simulink model "test_quadruped_troting"  (Simulink 9.2)
settings: Solver=VariableStepDiscrete  StartTime=0.0  StopTime=12  FixedStep=0.001  MaxStep=0.001  RelTol=1e-10  EnableMultiTasking=on
values from neighbouring files (symbols this model uses):
  Output_file_n = r_temp___(2)    [quadruped.m]
  Plant_inputs_num = r_temp___(1)    [quadruped.m]
  Plant_outputs_num = r_temp___(1)    [quadruped.m]
  RecurDyn_model_n = r_temp___(2)    [quadruped.m]
undefined symbols (not defined in the file): Matlab_version, Output_File, RecurDyn, RecurDyn_controltimestep, RecurDyn_model
(part 2 of 2)

== matlab function Subsystem/左前腿力//位控制单元 ==
  data: Th1 input double; qd input double; q input double; dot_qd input double; dot_q input double; LegMode input double; Fwd input double; Fwf input double; tau1 output double; Fr output double; Fe output double
function [tau1,Fr, Fe]  = SLC(Th1,qd,q,dot_qd,dot_q,LegMode, Fwd,Fwf)

%% 关节角度、足端广义坐标以及雅克比矩阵的计算
th11=Th1(1);
th12=Th1(2);
th13=Th1(3);

% 单腿连杆参数
L1 = 0.35*sqrt(2);
L2 = 0.35*sqrt(2);
R3 = 0.06;

% Jacobian Matrix
J1 = [ -L1*sin(th11 - th12),                   L2*sin(th12) + L1*sin(th11 - th12),                      0;...
          -L1*cos(th11 - th12)*cos(th13), -cos(th13)*(L2*cos(th12) - L1*cos(th11 - th12)), sin(th13)*(L2*sin(th12) + L1*sin(th11 - th12));...
          -L1*cos(th11 - th12)*sin(th13),  -sin(th13)*(L2*cos(th12) - L1*cos(th11 - th12)),  - cos(th13)*(L2*sin(th12) + L1*sin(th11 - th12))];

%% 初始化
 Fr=zeros(3,1);
 Fe = Fwf(1:3);    % 左前腿的足端接触力
 Fd = Fwd(1:3);
 
tau1=zeros(3,1);

%% 单腿力/位控制模式
y = LegMode;
switch(y)
%%%%%%%%%%%%%%%%%%%%%%%%%%%%%
    case 2      % 单腿支撑
        
%        p = diag([2.0  2.0  2.0]);       
%        p = diag([1.5  1.5  1.5]);
%        p = diag([1.4  1.4  1.4]);
%        p = diag([1.3  1.3  1.3]);
%        p = diag([1.2  1.2  1.2]);
       p = diag([1.1  1.1  1.1]);
%        p = diag([1.0  1.0  1.0]);
%        p = diag([0.9  0.9  0.9]);
%        p = diag([0.8  0.8  0.8]);
%        p = diag([0.7  0.7  0.7]);
%        p = diag([0.6  0.6  0.6]);
%        p = diag([0.5  0.5  0.5]);

       F=p*(Fd-Fe);
       Fr=Fd;
       
       tauf=J1'*(F+[0 Fe(2) 0]');
       tau1= -tauf;

%%%%%%%%%%%%%%%%%%%%%%%%%%%%%
    case 1    % 单腿摆动
        kp = diag([7500 7500 7500]);
        kd = diag([120 120 120]);
        
        Fr=zeros(3,1);
        tau1=J1'*(kp*(qd-q)+kd*(dot_qd-dot_q)); 
        
%%%%%%%%%%%%%%%%%%%%%%%%%%%%%
    case 0    % 落后着地
        kp = diag([1000 1500 1000]);
        kd = diag([20 30 20]);
        
        % 在y方向上补偿0.01m
        qd1= qd+[0;-0.01;0];     
        Fr=zeros(3,1);
        tau1=J1'*(kp*(qd1-q)+kd*(dot_qd-dot_q));

%%%%%%%%%%%%%%%%%%%%%%%%%%%%%
     case 3    % 提前着地
      
%        p = diag([1.2  1.2  1.2]);
       p = diag([0.8  0.8  0.8]);
       % y方向零力控制
       Fd=[0;5;0];
       F=p*(Fd-Fe);
       Fr=Fd;
       
       tauf=J1'*(F+[0 Fe(2) 0]');
       tau1=-tauf; 
end

%% 考虑实际情况：输出力矩限幅
Tmax = 500;

if tau1(1)>=Tmax
    tau1(1)=Tmax;
end
if tau1(1)<=-Tmax
    tau1(1)=-Tmax;
end
    
if tau1(2)>=Tmax
    tau1(2)=Tmax;
end
if tau1(2)<=-Tmax
    tau1(2)=-Tmax;
end
    
if tau1(3)>=Tmax
    tau1(3)=Tmax;
end
if tau1(3)<=-Tmax
    tau1(3)=-Tmax;
end

end

== matlab function 信号选择器 ==
  data: TipPos input double; HipPos output double
function HipPos  = SS(TipPos)

%% 
HipPos = TipPos(1:12);


end

== matlab function Subsystem/States Machine ==
  data: TorsoPosuture input double; VCoM input double; TipPos input double; TipForce input double; Time input double; RobotStates output double
function RobotStates   = StateMachine(TorsoPosuture, VCoM, TipPos, TipForce, Time)

% 状态机：根据当前机器人本体的状态变量 以及 足端接触力信息（作为开关量使用）， 判断并记录机器人某一特定状态及其对应的时刻
% BY ZPP
% 20171124

% TorsoPosuture：1*6（分别对应本体在世界坐标系的位置和姿态信息）
% TipForce：1*12（分别对应 左前/右前/左后/右后的足端三维力信息）
% Time：仿真时间

% RobotStates：1*35

%% 设置仿真状态初值
HipPos = TipPos(1:12);
if Time <= 0.001
    TorsoPosuture = [0; 0.70; 0;0;0;0];
    VCoM = zeros(6,1);
    HipPos = [0;-0.70;-0.0; 0;-0.70;+0.0; 0;-0.70;-0.0; 0;-0.70;+0.0];
    TipForce = zeros(12,1);
end

%% 声明局部静态变量
% 分别判断并记录四条腿TouchDown事件发生的时间点
persistent TDpoint_old1
persistent TDpoint_new1
persistent TDpoint_old2
persistent TDpoint_new2
persistent TDpoint_old3
persistent TDpoint_new3
persistent TDpoint_old4
persistent TDpoint_new4

% 分别判断并记录四条腿LiftOff事件发生的时间点
persistent LOpoint_old1
persistent LOpoint_new1
persistent LOpoint_old2
persistent LOpoint_new2
persistent LOpoint_old3
persistent LOpoint_new3
persistent LOpoint_old4
persistent LOpoint_new4

% 分别判断并记录四条腿TouchDown事件状态
persistent Swg_Sup_old1
persistent Swg_Sup_new1
persistent Swg_Sup_old2
persistent Swg_Sup_new2
persistent Swg_Sup_old3
persistent Swg_Sup_new3
persistent Swg_Sup_old4
persistent Swg_Sup_new4

% 2017/11/13增加 分别记录四条腿LiffOff事件发生时足端在髋部坐标系下的位置
persistent LOHx1_old  LOHy1_old  LOHz1_old
persistent LOHx2_old  LOHy2_old  LOHz2_old
persistent LOHx3_old  LOHy3_old  LOHz3_old
persistent LOHx4_old  LOHy4_old  LOHz4_old

persistent LOHx1_new  LOHy1_new  LOHz1_new
persistent LOHx2_new  LOHy2_new  LOHz2_new
persistent LOHx3_new  LOHy3_new  LOHz3_new
persistent LOHx4_new  LOHy4_new  LOHz4_new

% 记录本体竖直方向起跳高度以及起跳速度（所谓起跳，即四条腿均离地的那一个时刻对应的本体竖直方向高度与速度）
persistent LOTV_old
persistent LOTV_new
persistent LOTP_old
persistent LOTP_new

persistent NumTDL_old
persistent NumTDL_new

%  2017/7/19 增加  %%%%%%%%%%%%%%%%%%%%%%%%%%%%%%%%%%%
% 四足力分配模式选择（对于对角弹跳，则在【1,4】和【2,3】支撑之间选择）
persistent ForceDistMode_new
persistent ForceDistMode_old

% 2017/11/17 增加 记录力分配模式切换时间
persistent FDMSP_new
persistent FDMSP_old


% 本体在竖直方向上的位置与速度
persistent PYf_new
persistent PYf_old

% 2017/11/16新增
persistent VYf_new
persistent VYf_old

% 限制竖直方向上本体加速度切换的次数
persistent NumAccSwitch_new
persistent NumAccSwitch_old

%%%%%%%%%%%%%%%%%%%%%%%%%%%%%%%%%%%%%%%%%%%%%%

 % 变量初始化 %%%%%%%%%%%%%%%%%%%%%%%%%%%%%%%%%%%%%%
if isempty(LOTV_old)
    LOTV_old = 0;
end
if isempty(LOTV_new)
    LOTV_new = 0;
end
if isempty(LOTP_old)
    LOTP_old = 0;
end
 if isempty(LOTP_new)
    LOTP_new = 0;
 end
 
 
if isempty(NumTDL_old)
    NumTDL_old = 0;
end
 if isempty(NumTDL_new)
    NumTDL_new = 0;
end
 

if isempty(TDpoint_old1)
    TDpoint_old1 = 0;
end
if isempty(TDpoint_new1)
    TDpoint_new1 = 0;
end
if isempty(TDpoint_old2)
    TDpoint_old2 = 0;
end
if isempty(TDpoint_new2)
    TDpoint_new2 = 0;
end
if isempty(TDpoint_old3)
    TDpoint_old3 = 0;
end
if isempty(TDpoint_new3)
    TDpoint_new3 = 0;
end
if isempty(TDpoint_old4)
    TDpoint_old4 = 0;
end
if isempty(TDpoint_new4)
    TDpoint_new4 = 0;
end


if isempty(LOpoint_old1)
    LOpoint_old1 = 0;
end
if isempty(LOpoint_new1)
    LOpoint_new1 = 0;
end
if isempty(LOpoint_old2)
    LOpoint_old2 = 0;
end
if isempty(LOpoint_new2)
    LOpoint_new2 = 0;
end
if isempty(LOpoint_old3)
    LOpoint_old3 = 0;
end
if isempty(LOpoint_new3)
    LOpoint_new3 = 0;
end
if isempty(LOpoint_old4)
    LOpoint_old4 = 0;
end
if isempty(LOpoint_new4)
    LOpoint_new4 = 0;
end

%%%%%%%%%%%%%%%%%%%%%%%%%
if isempty(LOHx1_old)
    LOHx1_old = 0;
end
if isempty(LOHy1_old)
    LOHy1_old = 0;
end
if isempty(LOHz1_old)
    LOHz1_old = 0;
end

if isempty(LOHx2_old)
    LOHx2_old = 0;
end
if isempty(LOHy2_old)
    LOHy2_old = 0;
end
if isempty(LOHz2_old)
    LOHz2_old = 0;
end

if isempty(LOHx3_old)
    LOHx3_old = 0;
end
if isempty(LOHy3_old)
    LOHy3_old = 0;
end
if isempty(LOHz3_old)
    LOHz3_old = 0;
end

if isempty(LOHx4_old)
    LOHx4_old = 0;
end
if isempty(LOHy4_old)
    LOHy4_old = 0;
end
if isempty(LOHz4_old)
    LOHz4_old = 0;
end

%%%%

if isempty(LOHx1_new)
    LOHx1_new = 0;
end
if isempty(LOHy1_new)
    LOHy1_new = 0;
end
if isempty(LOHz1_new)
    LOHz1_new = 0;
end

if isempty(LOHx2_new)
    LOHx2_new = 0;
end
if isempty(LOHy2_new)
    LOHy2_new = 0;
end
if isempty(LOHz2_new)
    LOHz2_new = 0;
end

if isempty(LOHx3_new)
    LOHx3_new = 0;
end
if isempty(LOHy3_new)
    LOHy3_new = 0;
end
if isempty(LOHz3_new)
    LOHz3_new = 0;
end

if isempty(LOHx4_new)
    LOHx4_new = 0;
end
if isempty(LOHy4_new)
    LOHy4_new = 0;
end
if isempty(LOHz4_new)
    LOHz4_new = 0;
end

%%%%%%%%%%%%%%%%%%%%%%%%%

if isempty(Swg_Sup_old1)
    Swg_Sup_old1 = 0;
end
if isempty(Swg_Sup_new1)
    Swg_Sup_new1 = 0;
end
if isempty(Swg_Sup_old2)
    Swg_Sup_old2 = 0;
end
if isempty(Swg_Sup_new2)
    Swg_Sup_new2 = 0;
end
if isempty(Swg_Sup_old3)
    Swg_Sup_old3 = 0;
end
if isempty(Swg_Sup_new3)
    Swg_Sup_new3 = 0;
end
if isempty(Swg_Sup_old4)
    Swg_Sup_old4 = 0;
end
if isempty(Swg_Sup_new4)
    Swg_Sup_new4 = 0;
end


if isempty(ForceDistMode_new)
    ForceDistMode_new = 0;         % 【1】为奇数，表示为【1,4】支撑
end
if isempty(ForceDistMode_old)
    ForceDistMode_old = 0;         % 【1】为奇数，表示为【1,4】支撑
end
if isempty(FDMSP_new)
    FDMSP_new = 0;        
end
if isempty(FDMSP_old)
    FDMSP_old = 0;        
end




if isempty(PYf_new)
    PYf_new = 0;
end
if isempty(PYf_old)
    PYf_old = 0;
end

if isempty(VYf_new)
    VYf_new = 0;
end
if isempty(VYf_old)
    VYf_old = 0;
end

if isempty(NumAccSwitch_new)
    NumAccSwitch_new = 0;
end
if isempty(NumAccSwitch_old)
    NumAccSwitch_old = 0;
end


% 更新并存储上一周期和当前周期的状态值 %%%%%%%%%%%%%%%%%%%%%%%%%
lotp_old = LOTP_new;
LOTP_old = lotp_old;
lotv_old = LOTV_new;
LOTV_old = lotv_old;

numtdl_old = NumTDL_new;
NumTDL_old = numtdl_old;



tdp_old1 = TDpoint_new1;
TDpoint_old1 = tdp_old1;
tdp_old2 = TDpoint_new2;
TDpoint_old2 = tdp_old2;
tdp_old3 = TDpoint_new3;
TDpoint_old3 = tdp_old3;
tdp_old4 = TDpoint_new4;
TDpoint_old4 = tdp_old4;

lop_old1 = LOpoint_new1;
LOpoint_old1 = lop_old1;
lop_old2 = LOpoint_new2;
LOpoint_old2 = lop_old2;
lop_old3 = LOpoint_new3;
LOpoint_old3 = lop_old3;
lop_old4 = LOpoint_new4;
LOpoint_old4 = lop_old4;

%%%%%%%%%%%%%%%%%%%%%%%%
lohx1_old = LOHx1_new;
LOHx1_old = lohx1_old;
lohy1_old = LOHy1_new;
LOHy1_old = lohy1_old;
lohz1_old = LOHz1_new;
LOHz1_old = lohz1_old;

lohx2_old = LOHx2_new;
LOHx2_old = lohx2_old;
lohy2_old = LOHy2_new;
LOHy2_old = lohy2_old;
lohz2_old = LOHz2_new;
LOHz2_old = lohz2_old;

lohx3_old = LOHx3_new;
LOHx3_old = lohx3_old;
lohy3_old = LOHy3_new;
LOHy3_old = lohy3_old;
lohz3_old = LOHz3_new;
LOHz3_old = lohz3_old;

lohx4_old = LOHx4_new;
LOHx4_old = lohx4_old;
lohy4_old = LOHy4_new;
LOHy4_old = lohy4_old;
lohz4_old = LOHz4_new;
LOHz4_old = lohz4_old;

%%%%%%%%%%%%%%%%%%%%%%%%

swtotd_old1 = Swg_Sup_new1;
Swg_Sup_old1 = swtotd_old1;
swtotd_old2 = Swg_Sup_new2;
Swg_Sup_old2 = swtotd_old2;
swtotd_old3 = Swg_Sup_new3;
Swg_Sup_old3 = swtotd_old3;
swtotd_old4 = Swg_Sup_new4;
Swg_Sup_old4 = swtotd_old4;


ForceDM_old = ForceDistMode_new;
ForceDistMode_old = ForceDM_old;

fdmsp_old = FDMSP_new;
FDMSP_old = fdmsp_old;

PY_old = PYf_new;
PYf_old = PY_old;

VY_old = VYf_new;
VYf_old = VY_old;

numaccsw_old = NumAccSwitch_new;
NumAccSwitch_old = numaccsw_old;


%% 根据足端力初步判断触地状态(依此为左前/右前/左后/右后腿)  %%%%%%%%%%%%%%%%%%%%%
thre = 1;
LegState1 = (((abs(TipForce(1)))>=thre) || ((abs(TipForce(2)))>=thre) || ((abs(TipForce(3)))>=thre));  
LegState2 = (((abs(TipForce(4)))>=thre) || ((abs(TipForce(5)))>=thre) || ((abs(TipForce(6)))>=thre));  
LegState3 = (((abs(TipForce(7)))>=thre) || ((abs(TipForce(8)))>=thre) || ((abs(TipForce(9)))>=thre));  
LegState4 = (((abs(TipForce(10)))>=thre) || ((abs(TipForce(11)))>=thre) || ((abs(TipForce(12)))>=thre));  


%% 状态更新 %%%%%%%%%%%%%%%%%%%%%%%%%%%%%%%%%%%%%%%%%%%%%%

% 左前腿 %%%%%%%%%%%%%%%%%%%%%%%%%%%%%%%%%%%%%%%%%
Swg_Sup_new1 = double(LegState1);
if (Swg_Sup_new1==1) && (Swg_Sup_old1==0)
    % 由摆动向支撑切换，TouchDown事件发生的时刻得到更新
    TDpoint_new1 = Time;
     % 更新当前时刻机器人的触地状态为支撑状态
    Swg_Sup_new1 = 1;
    if ((TDpoint_new1-TDpoint_old1)<=0.05) || ((TDpoint_new1-LOpoint_new1)<=0.05)
    % 排除机器人触地瞬间在支撑期与摆动期之间高频切换（20Hz以上）
    % 否则不发生任何状态更新
    TDpoint_new1 = TDpoint_old1;
    Swg_Sup_new1 = Swg_Sup_old1;
    end
    % 但是 LiffOff 事件发生的时刻不更新
    LOpoint_new1 = LOpoint_old1;
    
elseif(Swg_Sup_new1==0) && (Swg_Sup_old1==1) 
% 同理，由支撑向摆动切换，LiffOff 事件发生的时刻得到更新
    LOpoint_new1 = Time;
    % 更新当前时刻机器人的触地状态为摆动状态
    Swg_Sup_new1 = 0;
    
    if ((LOpoint_new1-LOpoint_old1)<=0.05) || ((LOpoint_new1-TDpoint_new1)<=0.05)
        LOpoint_new1 = LOpoint_old1;
        Swg_Sup_new1 = Swg_Sup_old1;  
    end
    % 但是 TouchDown 事件发生的时刻不更新
    TDpoint_new1 = TDpoint_old1;
 
else
    % 否则不发生任何状态更新
    TDpoint_new1 = TDpoint_old1;
    LOpoint_new1 = LOpoint_old1;
    Swg_Sup_new1 = Swg_Sup_old1;  
end


% 右前腿 %%%%%%%%%%%%%%%%%%%%%%%%%%%%%%%%%%%%%%%%%
Swg_Sup_new2 = double(LegState2);
if (Swg_Sup_new2==1) && (Swg_Sup_old2==0)
    % 由摆动向支撑切换，TouchDown事件发生的时刻得到更新
    TDpoint_new2 = Time;
     % 更新当前时刻机器人的触地状态为支撑状态
    Swg_Sup_new2 = 1;
    if ((TDpoint_new2-TDpoint_old2)<=0.05) || ((TDpoint_new2-LOpoint_new2)<=0.05)
    % 排除机器人触地瞬间在支撑期与摆动期之间高频切换（100Hz以上）
    % 否则不发生任何状态更新
    TDpoint_new2 = TDpoint_old2;
    Swg_Sup_new2 = Swg_Sup_old2;
    end
    % 但是 LiffOff 事件发生的时刻不更新
    LOpoint_new2 = LOpoint_old2;
    
elseif(Swg_Sup_new2==0) && (Swg_Sup_old2==1) 
% 同理，由支撑向摆动切换，LiffOff 事件发生的时刻得到更新
    LOpoint_new2 = Time;
    % 更新当前时刻机器人的触地状态为摆动状态
    Swg_Sup_new2 = 0;
    
    if ((LOpoint_new2-LOpoint_old2)<=0.05) || ((LOpoint_new2-TDpoint_new2)<=0.05)
        LOpoint_new2 = LOpoint_old2;
        Swg_Sup_new2 = Swg_Sup_old2;  
    end
    % 但是 TouchDown 事件发生的时刻不更新
    TDpoint_new2 = TDpoint_old2;
 
else
    % 否则不发生任何状态更新
    TDpoint_new2 = TDpoint_old2;
    LOpoint_new2 = LOpoint_old2;
    Swg_Sup_new2 = Swg_Sup_old2;  
end

% 左后腿 %%%%%%%%%%%%%%%%%%%%%%%%%%%%%%%%%%%%%%%%%
Swg_Sup_new3 = double(LegState3);
if (Swg_Sup_new3==1) && (Swg_Sup_old3==0)
    % 由摆动向支撑切换，TouchDown事件发生的时刻得到更新
    TDpoint_new3 = Time;
     % 更新当前时刻机器人的触地状态为支撑状态
    Swg_Sup_new3 = 1;
    if ((TDpoint_new3-TDpoint_old3)<=0.05) || ((TDpoint_new3-LOpoint_new3)<=0.05)
    % 排除机器人触地瞬间在支撑期与摆动期之间高频切换（20Hz以上）
    % 否则不发生任何状态更新
    TDpoint_new3 = TDpoint_old3;
    Swg_Sup_new3 = Swg_Sup_old3;
    end
    % 但是 LiffOff 事件发生的时刻不更新
    LOpoint_new3 = LOpoint_old3;
    
elseif(Swg_Sup_new3==0) && (Swg_Sup_old3==1) 
% 同理，由支撑向摆动切换，LiffOff 事件发生的时刻得到更新
    LOpoint_new3 = Time;
    % 更新当前时刻机器人的触地状态为摆动状态
    Swg_Sup_new3 = 0;
    
    if ((LOpoint_new3-LOpoint_old3)<=0.05) || ((LOpoint_new3-TDpoint_new3)<=0.05)
        LOpoint_new3 = LOpoint_old3;
        Swg_Sup_new3 = Swg_Sup_old3;  
    end
    % 但是 TouchDown 事件发生的时刻不更新
    TDpoint_new3 = TDpoint_old3;
 
else
    % 否则不发生任何状态更新
    TDpoint_new3 = TDpoint_old3;
    LOpoint_new3 = LOpoint_old3;
    Swg_Sup_new3 = Swg_Sup_old3;  
end

% 右后腿%%%%%%%%%%%%%%%%%%%%%%%%%%%%%%%%%%%%%%%%%%%
Swg_Sup_new4 = double(LegState4);
if (Swg_Sup_new4==1) && (Swg_Sup_old4==0)
    % 由摆动向支撑切换，TouchDown事件发生的时刻得到更新
    TDpoint_new4 = Time;
     % 更新当前时刻机器人的触地状态为支撑状态
    Swg_Sup_new4 = 1;
    if ((TDpoint_new4-TDpoint_old4)<=0.05) || ((TDpoint_new4-LOpoint_new4)<=0.05)
    % 排除机器人触地瞬间在支撑期与摆动期之间高频切换（20Hz以上）
    % 否则不发生任何状态更新
    TDpoint_new4 = TDpoint_old4;
    Swg_Sup_new4 = Swg_Sup_old4;
    end
    % 但是 LiffOff 事件发生的时刻不更新
    LOpoint_new4 = LOpoint_old4;
    
elseif(Swg_Sup_new4==0) && (Swg_Sup_old4==1) 
% 同理，由支撑向摆动切换，LiffOff 事件发生的时刻得到更新
    LOpoint_new4 = Time;
    % 更新当前时刻机器人的触地状态为摆动状态
    Swg_Sup_new4 = 0;
    
    if ((LOpoint_new4-LOpoint_old4)<=0.05) || ((LOpoint_new4-TDpoint_new4)<=0.05)
        LOpoint_new4 = LOpoint_old4;
        Swg_Sup_new4 = Swg_Sup_old4;  
    end
    % 但是 TouchDown 事件发生的时刻不更新
    TDpoint_new4 = TDpoint_old4;
 
else
    % 否则不发生任何状态更新
    TDpoint_new4 = TDpoint_old4;
    LOpoint_new4 = LOpoint_old4;
    Swg_Sup_new4 = Swg_Sup_old4;  
end
%%%%%%%%%%%%%%%%%%%%%%%%%%%%%%%%%%%%%%%%%%%%%%%%
% Swg2Sup_old = [Swg_Sup_old1; Swg_Sup_old2; Swg_Sup_old3; Swg_Sup_old4];
Swg2Sup = [Swg_Sup_new1; Swg_Sup_new2; Swg_Sup_new3; Swg_Sup_new4];
TDP = [TDpoint_new1; TDpoint_new2; TDpoint_new3; TDpoint_new4];
LOP = [LOpoint_new1; LOpoint_new2; LOpoint_new3; LOpoint_new4];

% 稳定触地腿的数目
NumTDL = sum(sum(Swg2Sup));
% numtdl_old =  sum(sum(Swg2Sup_old));

%% 2017/11/16 限制竖直方向上本体加速度切换的次数
VYf_new = VCoM(2);
if (VYf_new >=0.40) && (VYf_old< 0.40) && (VYf_old>0.00)     % 【0.5m/s】 为本体在竖直方向上的期望起跳速度
    % 若达到期望起跳速度则切换
    NumAccSwitch_new = NumAccSwitch_old +1;
%     NumAccSwitch_new = NumAccSwitch_new
else
    % 否则不更新
    NumAccSwitch_new = NumAccSwitch_old;
end
% 进入四足腾空期，则清零
NumTDL_new = NumTDL;
if (NumTDL_new == 0)
    NumAccSwitch_new = 0;
    NumAccSwitch_old = 0;
end
numaccsw = NumAccSwitch_new;
    

%% 记录起跳时刻本体在竖直方向上的高度和速度
VyCoM = VCoM(2);
PYf = TorsoPosuture(2);

NumTDL_new = NumTDL;
% LOTP_new = PYf;
% LOTV_new = VyCoM;

if (NumTDL_new == 0) && ((NumTDL_old==2) || (NumTDL_old==1))
    % 由对角支撑期进入四足腾空期
    LOTP_new = PYf;
    LOTV_new = VyCoM;
else
    LOTP_new = LOTP_old;
    LOTV_new = LOTV_old;    
end

LOTPy = LOTP_new;
LOTVy = LOTV_new;


%% 力分配模式切换  以及 LiffOff 事件发生时刻足端在髋部坐标系下的位置

PYf_new = PYf;

if (PYf_new>=0.65) && (PYf_old<0.65)  % 【0.65】 表示腿长在【0.75m】的时候本体腾空
    % 完成一个弹跳周期进入腾空期，则四足机器人对角腿支撑进行交换，力分配模式变量得到更新
    ForceDistMode_new = ForceDistMode_old + 1;
    FDMSP_new = Time;
    % 若完成一次弹跳，则加速度切换次数清零

    %%%%%%%%%%%%%%%%%%%%%%%%%%%%%%%%%%%%%%%%%%%%%%%%%
    temp = mod(ForceDistMode_new,2);    % 奇数表示当前进入【1,4】腿支撑，偶数表示当前进入【2,3】腿支撑
    if (temp==0)  
        % Update【1,4】
        LOHx1_new = HipPos(1);  LOHy1_new = HipPos(2);  LOHz1_new = HipPos(3);
        LOHx4_new = HipPos(10);  LOHy4_new = HipPos(11);  LOHz4_new = HipPos(12);
        % maintain【2,3】
        LOHx2_new = LOHx2_old;  LOHy2_new = LOHy2_old;  LOHz2_new = LOHz2_old;
        LOHx3_new = LOHx3_old;  LOHy3_new = LOHy3_old;  LOHz3_new = LOHz3_old;
    else
        % Update【2,3】
        LOHx2_new = HipPos(4);  LOHy2_new = HipPos(5);  LOHz2_new = HipPos(6);
        LOHx3_new = HipPos(7);  LOHy3_new = HipPos(8);  LOHz3_new = HipPos(9);
        % maintain【1,4】
        LOHx1_new = LOHx1_old;  LOHy1_new = LOHy1_old;  LOHz1_new = LOHz1_old;
        LOHx4_new = LOHx4_old;  LOHy4_new = LOHy4_old;  LOHz4_new = LOHz4_old;
    end
    %%%%%%%%%%%%%%%%%%%%%%%%%%%%%%%%%%%%%%%%%%%%%%%%%    
else
    % 否则不更新
    ForceDistMode_new = ForceDistMode_old;
    FDMSP_new = FDMSP_old;
%     NumAccSwitch_new = NumAccSwitch_old;
    % maintain【1,4 & 2,3】
    LOHx1_new = LOHx1_old;  LOHy1_new = LOHy1_old;  LOHz1_new = LOHz1_old;
    LOHx4_new = LOHx4_old;  LOHy4_new = LOHy4_old;  LOHz4_new = LOHz4_old;
    LOHx2_new = LOHx2_old;  LOHy2_new = LOHy2_old;  LOHz2_new = LOHz2_old;
    LOHx3_new = LOHx3_old;  LOHy3_new = LOHy3_old;  LOHz3_new = LOHz3_old;
end

% 力分配模式：奇数为【1,4】腿支撑，偶数为【2,3】腿支撑
FDMode = mod(ForceDistMode_new,2);
FDMSP = FDMSP_new;
% 单腿LiffOff事件时刻足端在髋部坐标系下的位置
LOHipPos = [LOHx1_new; LOHy1_new; LOHz1_new; LOHx2_new; LOHy2_new; LOHz2_new; LOHx3_new; LOHy3_new; LOHz3_new; LOHx4_new; LOHy4_new; LOHz4_new];

%% 输出机器人状态信息
RobotStates = [TorsoPosuture; Swg2Sup; TDP; LOP; NumTDL; FDMode; LOTPy; LOTVy; LOHipPos; numaccsw;  FDMSP];

end

== matlab function Subsystem/LF足端位置规划/信号选择器 ==
  data: RS input double; TorsoPos output double
function TorsoPos  = SS(RS)

%% 选出机器人本体在世界坐标系中的位置以及姿态角
TorsoPos = RS(1:6);

end

== matlab function Subsystem/RF足端位置规划/rf ==
  data: Th2 output double; qd output double; q output double; ThVec input double; HipPos input double; RS input double; VCoM input double; Vxd input double; t input double; LegMode output double
function [Th2, qd, q, LegMode]  = fcn(ThVec, HipPos, RS, VCoM, Vxd, t)
% 定周期足端轨迹规划

%% 设置仿真状态初值
if t<=0.001
    ThVec = [pi/2;pi/4;0; pi/2;pi/4;0; pi/2;pi/4;0; pi/2;pi/4;0];
    HipPos = [0;-0.00;-0.0; 0;-0.70;+0.0; 0;-0.70;-0.0; 0;-0.70;+0.0];
    VCoM = zeros(6,1);
    RS = [0; 0.70; 0;0;0;0; zeros(13,1); 1;0;0; zeros(12,1); 0;  0];
end

%% 输出关节角度，足端广义坐标 (在髋部惯性系下)
x2 = HipPos(4);
y2 = HipPos(5);
z2 = HipPos(6);
q = [x2 y2 z2]';

% 右前腿的3个关节角
Th2 = ThVec(4:6);    

% 【1/4】腿腿长
y1 = HipPos(2);
y4 = HipPos(11);

%% 根据腿部状态选择单腿控制模式
%  LegMode = 0 ：支撑模式
%  LegMode = 1 ：摆动模式
%  LegMode = 2 ：落后着地
 %  LegMode = 3 ：提前着地
 
  % 支撑腿状态信息
%  Swg2Sup1 = RS(7);
%  Swg2Sup4 = RS(10);
  
Swg2Sup2 = RS(8);
NumTDL = RS(19);
ForceDM = RS(20);

% Y方向上的本体位置与速度
PY = RS(2);
% VY = VCoM(2);
% 设置期望的起跳高度以及起跳速度
Hlod = 0.65; % 对应腿长为0.75m
% Vlod = 0.5;


% 若进入【2/3】腿支撑模式
if (ForceDM==0)  
    if (Swg2Sup2==1)
        % 当前腿着地
        if (NumTDL==2) && (PY<Hlod)
        % 两足支撑且未达到起跳高度，进入对角腿支撑模式
            LegMode = 2;
        elseif(NumTDL<=2) && (PY>=Hlod)
        % 四足支撑且已经达到起跳高度，则缩腿进入单腿摆动模式
            LegMode = 1;
        else
        % 至少有一腿支撑，进入提前着地模式（零接触力控制）
            LegMode = 3;
        end
    
    else
        % 当前腿处于腾空期，则保持摆动模式，等待触地
        LegMode = 1;
    end
    
% 若 ForceDM==1，进入【1/4】腿支撑模式
else   
    % 则【2/3】腿始终处于摆动模式
    LegMode = 1;
end



%%  基于简单落足点选择的本体侧向速度控制策略  %%%%%%%%%%%%%%%%%%%%%%%%%%%%%%%%%%%%%%%

%%%  设置参数  %%%
vxd = Vxd;
vzd = 0;

vx = VCoM(1);
vz = VCoM(3);

%%%   起跳时刻【2/3】腿足端位置   %%%
lohx2 = RS(26);     lohz2 = RS(28);
% lohx3 = RS(29);     lohz3 = RS(31);

kx = 0.05;
kz = 0.04;

%%%   基于 Raibert 的算法计算落足点位置   %%%

%%%  根据前一个【2/3】腿对角支撑期估计下一个【1/4】腿对角支撑期的时长  %%%
t5 = min(RS(11),RS(14));      % 前一支撑期（t5）或下一支撑期（t9）【1/4】腿落足时刻
t6 = min(RS(15),RS(18));      % 前一支撑期（t6）或下一支撑期（t10）【1/4】腿抬腿时刻
t7 = min(RS(12),RS(13));      % 前一支撑期【2/3】腿落足时刻
t8 = min(RS(16),RS(17));      % 前一支撑期【2/3】腿抬腿时刻
FDMSP = RS(36);                   % 略大于t8或t10

%%%   对角腿支撑期时长计算或估计   %%%
supT_est = (FDMSP - t7)*(ForceDM==1) + (FDMSP - t5)*(ForceDM==0);
% 连续一个四足腾空期和一个对角支撑期时长计算或估计
swgsuppT_est = (FDMSP - t6)*(ForceDM==1) + (FDMSP - t8)*(ForceDM==0);


%%%  计算足端在【X/Z】方向上的落足点分量  %%%%
x2d = 0.5*supT_est*vx + kx*(vx-vxd);
z2d = 0.5*supT_est*vz + kz*(vz-vzd);

thre = 0.1;
if z2d>=thre
         z2d=thre;
     elseif z2d<=-thre;
         z2d=-thre;
end

%%%  三角函数规划足端在【X/Z】方向上的运动轨迹  %%%
if (t<FDMSP+swgsuppT_est) && (ForceDM==1)
    % 摆动阶段
    tempx2 = 0.5*(lohx2-x2d)*cos(pi*(t-FDMSP)/(swgsuppT_est))+0.5*(lohx2+ x2d);
    tempz2 = 0.5*(lohz2-z2d)*cos(pi*(t-FDMSP)/(swgsuppT_est))+0.5*(lohz2+ z2d);
else
    % 准备触地阶段
    tempx2 = x2d;
    tempz2 = z2d;    
end

% 
if (ForceDM==1)
    if (t5<=FDMSP)
        % 快速缩腿阶段
        tempy2 = -0.65;
    else
    % 快速摆动阶段：随动，使得在【1/4】腿支撑期间避免【2/3】腿支撑触地
        tempy2 = (0.5*(y1+y4)+0.05);
        if tempy2 <-0.70;
            tempy2 = -0.70;
        end
    end
else
    %  准备触地阶段
    tempy2 = -0.70;
end
qd = [tempx2; tempy2; tempz2];

% if Swg2Sup2==0
%     qd = [0; -0.70; +0.0];
%     LegMode = 1;
% else
%     LegMode = 2;
% end

% if (t<10)
%     qd = [0; -0.70; 0.05];
%     LegMode = 1;
% else
%     tempy2 = -0.70 + 0.01*(t-10);
%     qd = [0; tempy2; 0.05];
%     LegMode = 1;
% end

end

== matlab function Subsystem/RF足端位置规划/信号选择器 ==
  data: RS input double; TorsoPos output double
function TorsoPos  = SS(RS)

%% 选出机器人本体在世界坐标系中的位置以及姿态角
TorsoPos = RS(1:6);

end

== matlab function Subsystem/LH足端位置规划/lh ==
  data: Th3 output double; qd output double; q output double; ThVec input double; HipPos input double; RS input double; VCoM input double; Vxd input double; t input double; LegMode output double
function [Th3, qd, q, LegMode]  = fcn(ThVec, HipPos, RS, VCoM, Vxd, t)
% 定周期足端轨迹规划

%% 设置仿真状态初值
if t<=0.001
    ThVec = [pi/2;pi/4;0; pi/2;pi/4;0; pi/2;pi/4;0; pi/2;pi/4;0];
    HipPos = [0;-0.70;-0.0; 0;-0.70;+0.0; 0;-0.70;-0.0; 0;-0.70;+0.0];
    VCoM = zeros(6,1);
    RS = [0; 0.70; 0;0;0;0; zeros(13,1); 1;0;0; zeros(12,1); 0;  0];
end

%% 输出关节角度，足端广义坐标 (在髋部惯性系下)
x3 = HipPos(7);
y3 = HipPos(8);
z3 = HipPos(9);
q = [x3 y3 z3]';

% 左后腿的3个关节角
Th3 = ThVec(7:9);    

% 【1/4】腿腿长
y1 = HipPos(2);
y4 = HipPos(11);

%% 根据腿部状态选择单腿控制模式
%  LegMode = 0 ：支撑模式
%  LegMode = 1 ：摆动模式
%  LegMode = 2 ：落后着地
 %  LegMode = 3 ：提前着地
 
 % 支撑腿状态信息
%  Swg2Sup1 = RS(7);
%  Swg2Sup4 = RS(10);
 
Swg2Sup3 = RS(9);
NumTDL = RS(19);
ForceDM = RS(20);

% Y方向上的本体位置与速度
PY = RS(2);
% VY = VCoM(2);
% 设置期望的起跳高度以及起跳速度
Hlod = 0.65; % 对应腿长为0.75m
% Vlod = 0.5;

% 若进入【2/3】腿支撑模式
if (ForceDM==0)  
    if (Swg2Sup3==1)
        % 当前腿着地
        if (NumTDL==2) && (PY<Hlod)
        % 两足支撑且未达到起跳高度，进入对角腿支撑模式
            LegMode = 2;
        elseif(NumTDL<=2) && (PY>=Hlod)
        % 四足支撑且已经达到起跳高度，则缩腿进入单腿摆动模式
            LegMode = 1;
        else
        % 至少有一腿支撑，进入提前着地模式（零接触力控制）
            LegMode = 3;
        end
    
    else
        % 当前腿处于腾空期，则保持摆动模式，等待触地
        LegMode = 1;
    end
    
% 若 ForceDM==1，进入【1/4】腿支撑模式
else   
    % 则【2/3】腿始终处于摆动模式
    LegMode = 1;
end


%%  基于简单落足点选择的本体侧向速度控制策略  %%%%%%%%%%%%%%%%%%%%%%%%%%%%%%%%%%%%%%%

%%%  设置参数  %%%
vxd = Vxd;
vzd = 0;

vx = VCoM(1);
vz = VCoM(3);

%%%   起跳时刻【2/3】腿足端位置   %%%
% lohx2 = RS(26);     lohz2 = RS(28);
lohx3 = RS(29);     lohz3 = RS(31);

kx = 0.05;
kz = 0.04;

%%%   基于 Raibert 的算法计算落足点位置   %%%

%%%  根据前一个【2/3】腿对角支撑期估计下一个【1/4】腿对角支撑期的时长  %%%
t5 = min(RS(11),RS(14));      % 前一支撑期（t5）或下一支撑期（t9）【1/4】腿落足时刻
t6 = min(RS(15),RS(18));      % 前一支撑期（t6）或下一支撑期（t10）【1/4】腿抬腿时刻
t7 = min(RS(12),RS(13));      % 前一支撑期【2/3】腿落足时刻
t8 = min(RS(16),RS(17));      % 前一支撑期【2/3】腿抬腿时刻
FDMSP = RS(36);                   % 略大于t8或t10

%%%   对角腿支撑期时长计算或估计   %%%
supT_est = (FDMSP - t7)*(ForceDM==1) + (FDMSP - t5)*(ForceDM==0);
% 连续一个四足腾空期和一个对角支撑期时长计算或估计
swgsuppT_est = (FDMSP - t6)*(ForceDM==1) + (FDMSP - t8)*(ForceDM==0);


%%%  计算足端在【X/Z】方向上的落足点分量  %%%%
x3d = 0.5*supT_est*vx + kx*(vx-vxd);
z3d = 0.5*supT_est*vz + kz*(vz-vzd);

thre = 0.1;
if z3d>=thre
         z3d=thre;
     elseif z3d<=-thre;
         z3d=-thre;
end

%%%  三角函数规划足端在【X/Z】方向上的运动轨迹  %%%
if (t<FDMSP+swgsuppT_est)  && (ForceDM==1)
    % 摆动阶段
    tempx3 = 0.5*(lohx3-x3d)*cos(pi*(t-FDMSP)/(swgsuppT_est))+0.5*(lohx3+ x3d);
    tempz3 = 0.5*(lohz3-z3d)*cos(pi*(t-FDMSP)/(swgsuppT_est))+0.5*(lohz3+ z3d);
else
    % 准备触地阶段
    tempx3 = x3d;
    tempz3 = z3d;    
end

% 
if (ForceDM==1)
    if (t5<=FDMSP)
        % 快速缩腿阶段
        tempy3 = -0.65;
    else
    % 快速摆动阶段：随动，使得在【1/4】腿支撑期间避免【2/3】腿支撑触地
        tempy3 = (0.5*(y1+y4)+0.05);
        if tempy3 <-0.70;
            tempy3 = -0.70;
        end
    end
else
    %  准备触地阶段
    tempy3 = -0.70;
end
qd = [tempx3; tempy3; tempz3];

% if Swg2Sup3==0
%     qd = [0; -0.70; -0.0];
%     LegMode = 1;
% else
%     LegMode = 2;
% end

% if (t<10)
%     qd = [0; -0.70; -0.05];
%     LegMode = 1;
% else
%     qd = [0; -0.70; -0.05];
%     LegMode = 1;
% end

end

== matlab function Subsystem/LH足端位置规划/信号选择器 ==
  data: RS input double; TorsoPos output double
function TorsoPos  = SS(RS)

%% 选出机器人本体在世界坐标系中的位置以及姿态角
TorsoPos = RS(1:6);

end

== matlab function Subsystem/RH足端位置规划/rh ==
  data: Th4 output double; qd output double; q output double; ThVec input double; HipPos input double; RS input double; VCoM input double; Vxd input double; t input double; LegMode output double
function [Th4, qd, q, LegMode]  = fcn(ThVec, HipPos, RS, VCoM, Vxd, t)
% 定周期足端轨迹规划

%% 设置仿真状态初值
if t<=0.001
    ThVec = [pi/2;pi/4;0; pi/2;pi/4;0; pi/2;pi/4;0; pi/2;pi/4;0];
    HipPos = [0;-0.70;-0.0; 0;-0.70;+0.0; 0;-0.70;-0.0; 0;-0.70;+0.0];
    VCoM = zeros(6,1);
    RS = [0; 0.70; 0;0;0;0; zeros(13,1); 1;0;0; zeros(12,1); 0;  0];
end

%% 输出关节角度，足端广义坐标 (在髋部惯性系下)
x4 = HipPos(10);
y4 = HipPos(11);
z4 = HipPos(12);
q = [x4 y4 z4]';

% 右后腿的四个关节角
Th4 = ThVec(10:12);    

% 【2/3】腿腿长
y2 = HipPos(5);
y3 = HipPos(8);

%% 根据腿部状态选择单腿控制模式
%  LegMode = 0 ：支撑模式
%  LegMode = 1 ：摆动模式
%  LegMode = 2 ：落后着地
 %  LegMode = 3 ：提前着地
 
 % 支撑腿状态信息
% Swg2Sup2 = RS(8);
% Swg2Sup3 = RS(9);
 
Swg2Sup4 = RS(10);
NumTDL = RS(19);
ForceDM = RS(20);

% Y方向上的本体位置与速度
PY = RS(2);
% VY = VCoM(2);
% 设置期望的起跳高度以及起跳速度
Hlod = 0.65; % 对应腿长为0.75m
% Vlod = 0.5;

% 若进入【1/4】腿支撑模式
if (ForceDM==1)  
    if (Swg2Sup4==1)
        % 当前腿着地
        if (NumTDL==2) && (PY<Hlod)
        % 两足支撑且未达到起跳高度，进入对角腿支撑模式
            LegMode = 2;
        elseif(NumTDL<=2) && (PY>=Hlod)
        % 四足支撑且已经达到起跳高度，则缩腿进入单腿摆动模式
            LegMode = 1;
        else
        % 至少有一腿支撑，进入提前着地模式（零接触力控制）
            LegMode = 3;
        end
    
    else
        % 当前腿处于腾空期，则保持摆动模式，等待触地
        LegMode = 1;
    end
    
% 若 ForceDM==0，进入【2/3】腿支撑模式
else   
    % 则【1/4】腿始终处于摆动模式
    LegMode = 1;
end


%%  基于简单落足点选择的本体侧向速度控制策略  %%%%%%%%%%%%%%%%%%%%%%%%%%%%%%%%%%%%%%%

%%%  设置参数  %%%
vxd = Vxd;
vzd = 0;

vx = VCoM(1);
vz = VCoM(3);

%%%   起跳时刻【1/4】腿足端位置   %%%
% lohx1 = RS(23);     lohz1 = RS(25);
lohx4 = RS(32);     lohz4 = RS(34);

kx = 0.05;
kz = 0.04;

%%%   基于 Raibert 的算法计算落足点位置   %%%

%%%  根据前一个【1/4】腿对角支撑期估计下一个【2/3】腿对角支撑期的时长  %%%
t3 = min(RS(12),RS(13));      % 前一支撑期（t3）或下一支撑期（t7）【2/3】腿落足时刻
t4 = min(RS(16),RS(17));      % 前一支撑期（t4）或下一支撑期（t8）【2/3】腿抬腿时刻
t5 = min(RS(11),RS(14));      % 前一支撑期【1/4】腿落足时刻
t6 = min(RS(15),RS(18));      % 前一支撑期【1/4】腿抬腿时刻
FDMSP = RS(36);                   % 略大于t6或t8

%%%   对角腿支撑期时长计算或估计   %%%
supT_est = (FDMSP - t5)*(ForceDM==0) + (FDMSP - t3)*(ForceDM==1);
% 连续一个四足腾空期和一个对角支撑期时长计算或估计
swgsuppT_est = (FDMSP - t4)*(ForceDM==0) + (FDMSP - t6)*(ForceDM==1);


%%%  计算足端在【X/Z】方向上的落足点分量  %%%%
x4d = 0.5*supT_est*vx + kx*(vx-vxd);
z4d = 0.5*supT_est*vz + kz*(vz-vzd);

thre = 0.1;
if z4d>=thre
         z4d=thre;
     elseif z4d<=-thre;
         z4d=-thre;
end

%%%  三角函数规划足端在【X/Z】方向上的运动轨迹  %%%
if (t<FDMSP+swgsuppT_est) && (ForceDM==0)
    % 摆动阶段
    tempx4 = 0.5*(lohx4-x4d)*cos(pi*(t-FDMSP)/(swgsuppT_est))+0.5*(lohx4+ x4d);
    tempz4 = 0.5*(lohz4-z4d)*cos(pi*(t-FDMSP)/(swgsuppT_est))+0.5*(lohz4+ z4d);
else
    % 准备触地阶段
    tempx4 = x4d;
    tempz4 = z4d;    
end

% 
if (ForceDM==0)
    if (t3<=FDMSP)
        % 快速缩腿阶段
        tempy4 = -0.65;
    else
    % 快速摆动阶段：随动，使得在【2/3】腿支撑期间避免【1/4】腿支撑触地
        tempy4 = (0.5*(y2+y3)+0.05);
        if tempy4 <-0.70;
            tempy4 = -0.70;
        end
    end
else
    %  准备触地阶段
    tempy4 = -0.70;
end
qd = [tempx4; tempy4; tempz4];

% if Swg2Sup4==0
%     qd = [0; -0.70; +0.0];
%     LegMode = 1;
% else
%     LegMode = 2;
% end

% if (t<10)
%     qd = [0.2; -0.70; 0.05];
%     LegMode = 1;
% else
%     qd = [0.2; -0.70; 0.05];
%     LegMode = 1;
% end

end

== matlab function Subsystem/RH足端位置规划/信号选择器 ==
  data: RS input double; TorsoPos output double
function TorsoPos  = SS(RS)

%% 选出机器人本体在世界坐标系中的位置以及姿态角
TorsoPos = RS(1:6);

end

== matlab function Subsystem/LF足端位置规划/lf ==
  data: Th1 output double; qd output double; q output double; ThVec input double; HipPos input double; RS input double; VCoM input double; Vxd input double; t input double; LegMode output double
function [Th1, qd, q, LegMode]  = fcn(ThVec, HipPos, RS, VCoM, Vxd, t)
% 定周期足端轨迹规划

%% 设置仿真状态初值
if t<=0.001
    ThVec = [pi/2;pi/4;0; pi/2;pi/4;0; pi/2;pi/4;0; pi/2;pi/4;0];
    HipPos = [0;-0.70;-0.0; 0;-0.70;+0.0; 0;-0.70;-0.0; 0;-0.70;+0.0];
    VCoM = zeros(6,1);
    RS = [0; 0.70; 0;0;0;0; zeros(13,1); 1;0;0; zeros(12,1); 0;  0];
end

%% 输出关节角度，足端广义坐标 (在髋部惯性系下)
x1 = HipPos(1);
y1 = HipPos(2);
z1 = HipPos(3);
q = [x1 y1 z1]';

% 左前腿的3个关节角
Th1 = ThVec(1:3);    

% 【2/3】腿腿长（足端位置竖直方向分量）
y2 = HipPos(5);
y3 = HipPos(8);

%% 根据腿部状态选择单腿控制模式，并进行弹跳控制
%  LegMode = 0 ：落后着地
%  LegMode = 1 ：摆动模式
%  LegMode = 2 ：支撑模式
 %  LegMode = 3 ：提前着地

 % 支撑腿状态信息
% Swg2Sup2 = RS(8);
% Swg2Sup3 = RS(9);
 
Swg2Sup1 = RS(7);
NumTDL = RS(19);
ForceDM = RS(20);

% Y方向上的本体位置与速度
PY = RS(2);
% VY = VCoM(2);
% 设置期望的起跳高度以及起跳速度
Hlod = 0.65; % 对应腿长为0.75m
% Vlod = 0.5;

% 若进入【1/4】腿支撑模式
if (ForceDM==1)  
    if (Swg2Sup1==1)
        % 若当前腿着地
        if (NumTDL==2) && (PY<Hlod)
        % 两足支撑且未达到起跳高度，进入对角腿支撑模式
            LegMode = 2;
        elseif(NumTDL<=2) && (PY>=Hlod)
        % 两足支撑且已经达到起跳高度，则缩腿进入单腿摆动模式
            LegMode = 1;
        else
        % 至少有一腿支撑，进入提前着地模式（零接触力控制）
            LegMode = 3;
        end
    
    else
        % 当前腿处于腾空期，则保持摆动模式，等待触地
        LegMode = 1;
    end
    
% 若 ForceDM==0，进入【2/3】腿支撑模式
else   
    % 则【1/4】腿始终处于摆动模式
    LegMode = 1;
end


%%  基于简单落足点选择的本体侧向速度控制策略  %%%%%%%%%%%%%%%%%%%%%%%%%%%%%%%%%%%%%%%

%%%  设置参数  %%%
vxd = Vxd;
vzd = 0;

vx = VCoM(1);
vz = VCoM(3);

%%%   起跳时刻【1/4】腿足端位置   %%%
lohx1 = RS(23);     lohz1 = RS(25);
% lohx4 = RS(32);     lohz4 = RS(34);

kx = 0.05;
kz = 0.04;

%%%   基于 Raibert 的算法计算落足点位置   %%%

%%%  根据前一个【1/4】腿对角支撑期估计下一个【2/3】腿对角支撑期的时长  %%%
t3 = min(RS(12),RS(13));      % 前一支撑期（t3）或下一支撑期（t7）【2/3】腿落足时刻
t4 = min(RS(16),RS(17));      % 前一支撑期（t4）或下一支撑期（t8）【2/3】腿抬腿时刻
t5 = min(RS(11),RS(14));      % 前一支撑期【1/4】腿落足时刻
t6 = min(RS(15),RS(18));      % 前一支撑期【1/4】腿抬腿时刻
FDMSP = RS(36);                   % 略大于t6或t8

%%%   对角腿支撑期时长计算或估计   %%%
supT_est = (FDMSP - t5)*(ForceDM==0) + (FDMSP - t3)*(ForceDM==1);
% 连续一个四足腾空期和一个对角支撑期时长计算或估计
swgsuppT_est = (FDMSP - t4)*(ForceDM==0) + (FDMSP - t6)*(ForceDM==1);


%%%  计算足端在【X/Z】方向上的落足点分量  %%%%
x1d = 0.5*supT_est*vx + kx*(vx-vxd);
z1d = 0.5*supT_est*vz + kz*(vz-vzd);

thre = 0.1;
if z1d>=thre
         z1d=thre;
     elseif z1d<=-thre;
         z1d=-thre;
end

%%%  三角函数规划足端在【X/Z】方向上的运动轨迹  %%%
if (t<FDMSP+swgsuppT_est) && (ForceDM==0)
    % 摆动阶段
    tempx1 = 0.5*(lohx1-x1d)*cos(pi*(t-FDMSP)/(swgsuppT_est))+0.5*(lohx1+ x1d);
    tempz1 = 0.5*(lohz1-z1d)*cos(pi*(t-FDMSP)/(swgsuppT_est))+0.5*(lohz1+ z1d);
else
    % 准备触地阶段
    tempx1 = x1d;
    tempz1 = z1d;    
end

% 
if (ForceDM==0)
    if (t3<=FDMSP)
        % 快速缩腿阶段
        tempy1 = -0.65;
    else
    % 快速摆动阶段：随动，使得在【2/3】腿支撑期间避免【1/4】腿支撑触地
        tempy1 = (0.5*(y2+y3)+0.05);
        if tempy1 <-0.70;
            tempy1 = -0.70;
        end
    end
else
    %  准备触地阶段
    tempy1 = -0.70;
end
qd = [tempx1; tempy1; tempz1];

% if Swg2Sup1==0
%     qd = [0; -0.70; -0.0];
%     LegMode = 1;
% else
%     LegMode = 2;
% end

% if (t<10)
%     qd = [0; -0.70; -0.05];
%     LegMode = 1;
% else
%     qd = [0; -0.70; -0.05];
%     LegMode = 1;
% end

end
